simulink model "buckboost_working"  (R2021a)
settings: Solver=VariableStepAuto  StartTime=0.0  StopTime=1  RelTol=1e-3
libraries: spsSeriesRLCBranchLib x4, spsCurrentMeasurementLib x2, spsIGBTDiodeLib x2, spsDCVoltageSourceLib x1, spsPWMGeneratorDCDCLib x1, spsVoltageMeasurementLib x1, spspowerguiLib x1
settings Model: Creator=SRIPARNO  LastModifiedBy=kallol bhattacharyya
settings SolverCC: ZeroCrossAlgorithm=Adaptive
settings DebuggingCC: IgnoredZcDiagnostic=none

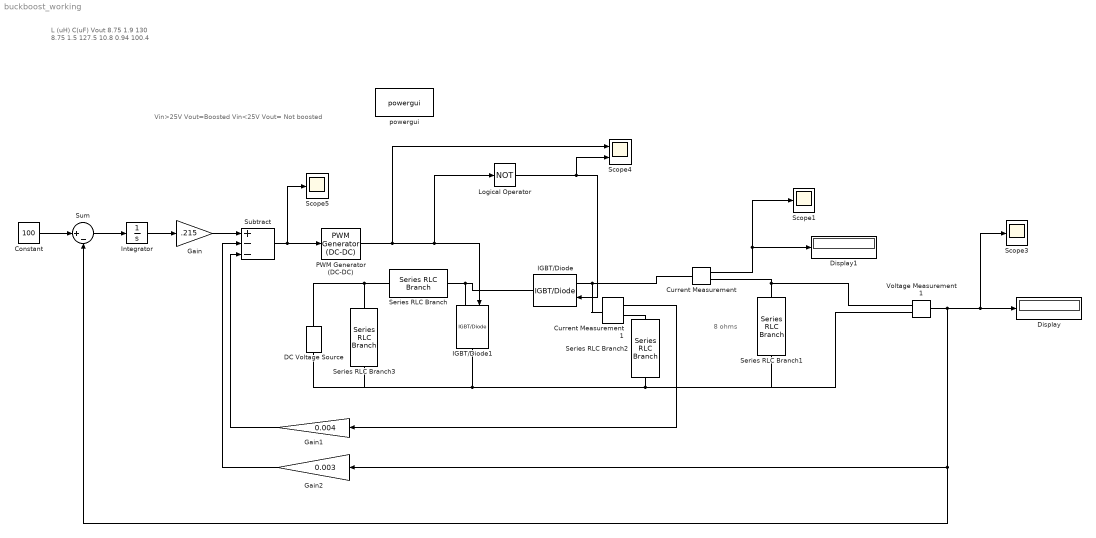
== system buckboost_working ==
  note: Vin>25V Vout=Boosted
      | Vin<25V Vout= Not boosted
  note: L (uH)         C(uF)          Vout
      | 8.75             1.9             130
      | 8.75             1.5              127.5
      | 10.8             0.94            100.4
  note: 8 ohms
  Constant : Constant  Value=100
  Current Measurement : spsCurrentMeasurementLib/Current Measurement  PhasorSimulation=off  OutputType=Complex  PSBequivalent=0
  Current Measurement1 : spsCurrentMeasurementLib/Current Measurement  PhasorSimulation=off  OutputType=Complex  PSBequivalent=0
  DC Voltage Source : spsDCVoltageSourceLib/DC Voltage Source  Amplitude=26  Measurements=None
  Display : Display
  Display1 : Display
  Gain : Gain  Gain=.215
  Gain1 : Gain  Gain=0.004
  Gain2 : Gain  Gain=0.003
  IGBT/Diode : spsIGBTDiodeLib/IGBT//Diode  Ron=1e-3  Rs=1e5  Cs=inf  Measurements=off
  IGBT/Diode1 : spsIGBTDiodeLib/IGBT//Diode  Ron=1e-3  Rs=1e5  Cs=inf  Measurements=off
  Integrator : Integrator
  Logical Operator : Logic  Operator=NOT  AllPortsSameDT=off  OutDataTypeStr=boolean
  PWM Generator (DC-DC) : spsPWMGeneratorDCDCLib/PWM Generator (DC-DC)  Fsw=25000  Ts=0
  Scope1 : Scope
  Scope3 : Scope
  Scope4 : Scope  NumInputPorts=2
  Scope5 : Scope
  Series RLC Branch : spsSeriesRLCBranchLib/Series RLC Branch  LConnTagsString=__new0  RConnTagsString=__new0  BranchType=L  Resistance=1  Inductance=1e-06  SetiL0=off  InitialCurrent=0  Capacitance=1e-6  Setx0=off  InitialVoltage=0  Measurements=None
  Series RLC Branch1 : spsSeriesRLCBranchLib/Series RLC Branch  LConnTagsString=__new0  RConnTagsString=__new0  BranchType=R  Resistance=50  Inductance=1e-3  SetiL0=off  InitialCurrent=0  Capacitance=1e-6  Setx0=off  InitialVoltage=0  Measurements=None
  Series RLC Branch2 : spsSeriesRLCBranchLib/Series RLC Branch  LConnTagsString=__new0  RConnTagsString=__new0  BranchType=C  Resistance=.001  Inductance=1e-3  SetiL0=off  InitialCurrent=0  Capacitance=.98e-03  Setx0=off  InitialVoltage=0  Measurements=None
  Series RLC Branch3 : spsSeriesRLCBranchLib/Series RLC Branch  LConnTagsString=__new0  RConnTagsString=__new0  BranchType=RC  Resistance=0.001  Inductance=400e-06  SetiL0=off  InitialCurrent=0  Capacitance=1.25e-6  Setx0=off  InitialVoltage=0  Measurements=None
  Subtract : Sum  Inputs=+--
  Sum : Sum  Inputs=|+-
  Voltage Measurement1 : spsVoltageMeasurementLib/Voltage Measurement  PhasorSimulation=off  OutputType=Complex  PSBequivalent=0
  powergui : spspowerguiLib/powergui  Priority=1  SimulationMode=Continuous  SampleTime=50e-6  frequency=60  Iterations=50  frequencyindice=0  Pbase=100e6  ErrMax=1e-4  UnitsV=kV  UnitsW=MW  buscounter=0  FunctionMessages=off  echomessages=off  EnableUseOfTLC=off  CurrentSourceSwitches=off  DisableSnubberDevices=off  DisableRonSwitches=off  DisableVfSwitches=off  DisplayEquations=off  AutomaticDiscreteSolvers=off  SolverType=Tustin/Backward Euler (TBE)  Interpol=off  ExternalGateDelay=off  methode=off  Ts=100  x0status=blocks  SPID=on  SwTol=0  HookPort=off  NonlinearTolerance=1e-4  nMaxIteration=100  ContinueOnMaxIteration=off  RestoreLinks=warning  ResistiveCurrentMeasurement=off  Frange=[0:2:500]  Ylog=off  Xlog=on  ShowGrid=off  save=off  variable=ZData  structure=0  ZoomFFT=off  StartTime=0.0  cycles=1  DisplayStyle=1  fundamental=60  FreqAxis=off  MaxFrequency=1000  frequencyindicesteady=1  RmsSteady=1  display=off
  wires:
  Current Measurement/1 -> Display1/1, Scope1/1
  Voltage Measurement1/1 -> Scope3/1, Display/1, Gain2/1, Sum/2
  Constant/1 -> Sum/1
  Sum/1 -> Integrator/1
  Integrator/1 -> Gain/1
  Gain/1 -> Subtract/1
  Gain1/1 -> Subtract/3
  Current Measurement1/1 -> Gain1/1
  Subtract/1 -> Scope5/1, PWM Generator (DC-DC)/1
  PWM Generator (DC-DC)/1 -> Scope4/1, Logical Operator/1, IGBT/Diode1/1
  Logical Operator/1 -> Scope4/2, IGBT/Diode/1
  Gain2/1 -> Subtract/2
  connections:
  Series RLC Branch2/RConn1 -- Series RLC Branch3/RConn1 -- DC Voltage Source/LConn1 -- IGBT/Diode1/RConn1 -- Series RLC Branch1/RConn1 -- Voltage Measurement1/LConn2
  Series RLC Branch1/LConn1 -- Current Measurement/RConn1 -- Voltage Measurement1/LConn1
  Series RLC Branch/RConn1 -- IGBT/Diode1/LConn1 -- IGBT/Diode/RConn1
  Current Measurement1/LConn1 -- IGBT/Diode/LConn1 -- Current Measurement/LConn1
  DC Voltage Source/RConn1 -- Series RLC Branch3/LConn1 -- Series RLC Branch/LConn1
  Current Measurement1/RConn1 -- Series RLC Branch2/LConn1
